simulink model "realsim"  (R2019b)
settings: Solver=VariableStepAuto  StartTime=0.0  StopTime=35  RelTol=1e-3
values from neighbouring files (symbols this model uses):
  d_den = [L*Je L*b+R*Je+kt*ke R*b]    [SystemModel.m]
  d_num = [L*r R*r]    [SystemModel.m]
  fd = fd_vec(1)    [SystemModel.m]
  p_den = [L*Je L*b+R*Je+kt*ke R*b]    [SystemModel.m]
  p_num = [kt]    [SystemModel.m]
  t_den = [1 tau]    [SystemModel.m]
  t_num = [tau]    [SystemModel.m]
  volt = volt_vec(i)    [SystemModel.m]
settings Model: Creator=keato  LastModifiedBy=keato

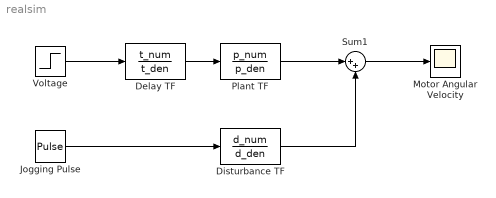
== system realsim ==
  Delay TF : TransferFcn  Numerator=t_num  Denominator=t_den
  Disturbance TF : TransferFcn  Numerator=d_num  Denominator=d_den
  Jogging Pulse : DiscretePulseGenerator  PulseType=Time based  Amplitude=fd  Period=1
  Motor Angular Velocity : Scope
  Plant TF : TransferFcn  Numerator=p_num  Denominator=p_den
  Sum1 : Sum  Inputs=|++
  Voltage : Step  After=volt  SampleTime=0
  wires:
  Voltage/1 -> Delay TF/1
  Delay TF/1 -> Plant TF/1
  Plant TF/1 -> Sum1/1
  Sum1/1 -> Motor Angular Velocity/1
  Disturbance TF/1 -> Sum1/2
  Jogging Pulse/1 -> Disturbance TF/1
